simulink model "IRB140"  (R2016b)
settings: Solver=ode113  StartTime=0.0  StopTime=40  RelTol=1e-3
(part 3 of 9)

== matlab function IRB140/PD controller1 ==
  data: theta_desired input; theta input; u output; thetad input
function u = fcn(theta_desired, theta, thetad)
e_theta = theta - theta_desired;

theta1 = theta(1);
theta2 = theta(2);
theta3 = theta(3);
theta4 = theta(4);
theta5 = theta(5);
theta6 = theta(6);

g = 9.81;

G1 = 0;
G2 = (g*(57*sin(theta2)*cos(theta3)*cos(theta4)*sin(theta5) + 57*sin(theta3)*cos(theta2)*cos(theta4)*sin(theta5) ...
    + 57*sin(theta2)*sin(theta3)*cos(theta5) + 3186*sin(theta2)*cos(theta3)*sin(theta4) ... 
    + 3186*sin(theta3)*cos(theta2)*sin(theta4) - 57*cos(theta2)*cos(theta3)*cos(theta5) + 418*sin(theta2)*sin(theta3) ... 
    - 418*cos(theta2)*cos(theta3) - 99072*sin(theta2)))/20000;
G3 = 57*(((-cos(theta5) - 22/3)*cos(theta3) + (1062*sin(theta3)*((19*cos(theta4)*sin(theta5))/1062 ...
    + sin(theta4)))/19)*cos(theta2) + ((cos(theta4)*sin(theta5) + (1062*sin(theta4))/19)*cos(theta3) ...
    + (cos(theta5) + 22/3)*sin(theta3))*sin(theta2))*g/20000;
G4 = -57*(sin(theta2)*sin(theta3) - cos(theta2)*cos(theta3))*g*(sin(theta4)*sin(theta5) - (1062*cos(theta4))/19)/20000;
G5 = 57*(cos(theta5)*(sin(theta2)*sin(theta3) - cos(theta2)*cos(theta3))*cos(theta4) ...
    + (cos(theta2)*sin(theta3) + sin(theta2)*cos(theta3))*sin(theta5))*g/20000;
G6 = 0;

G = [G1; G2; G3; G4; G5; G6];

Kp = diag([0.5 10 1 1 1 1])*100;
Kd = eye(6) * 10;
u = -Kp*e_theta - Kd*thetad + G;
